simulink model "slxcases"  (R2027a)
settings: Solver=VariableStepAuto
model workspace (MAT data in the model file):
  cfg.mode = 'fast'
  cfg.gain = 2
  flag = 1
  grid = [1  2  3; 4  5  6]
  inner = 7
  label = 'hello'
  names = {'alpha', 'beta'}
  span = 3
  tau = 0.25
undefined symbols (not defined in the file or in its folder): Ki, Kp
settings Model: DataDictionary=slxparams.sldd  Creator=weiwang  LastModifiedBy=weiwang

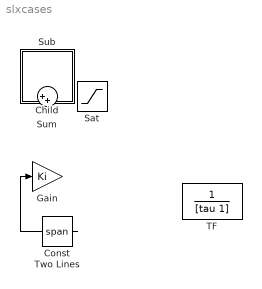
== system slxcases ==
  Child : ModelReference  ZOffset=3  ModelNameDialog=slx_child  ModelReferenceVersion=1.1
  Const : Constant  Value=Kp
  Gain : Gain  Gain=Ki
  Sat : Saturate  UpperLimit=Inf  LowerLimit=-Inf
  Sub : Subsystem  ZOffset=2
  Sum : Sum  Inputs=|++
  TF : TransferFcn  Denominator=[tau 1]
  Two Lines : Constant  ZOffset=1  Value=span
  wires:
  Const/1 -> Gain/1

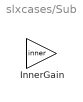
== system slxcases/Sub ==
  InnerGain : Gain  Gain=inner
